simulink model "Recharge"  (R2020a)
settings: Solver=FixedStepAuto  StartTime=0.0  StopTime=10.0  FixedStep=1e-3  RelTol=1e-3  EnableMultiTasking=on
settings Model: ExtModeTrigDuration=5  Creator=WinnieTrandinh  LastModifiedBy=WinnieTrandinh
settings OptimizationCC: EnhancedBackFolding=on  PassReuseOutputArgsAs=Individual arguments  ZeroExternalMemoryAtStartup=off  ZeroInternalMemoryAtStartup=off  MaxStackSize=64  OptimizeBlockOrder=speed  DifferentSizesBufferReuse=on  OptimizationCustomize=off  EfficientTunableParamExpr=on
settings DebuggingCC: ParameterTunabilityLossMsg=error
settings HardwareCC: ProdBitPerPointer=32  ProdBitPerSizeT=32  ProdBitPerPtrDiffT=32  ProdLargestAtomicInteger=Long  ProdLargestAtomicFloat=Double  ProdWordSize=32  ProdHWDeviceType=ARM Compatible->ARM Cortex
settings SFSimCC: MATLABDynamicMemAlloc=off
settings RTWCC: SystemTargetFile=ert.tlc  HardwareBoard=NXP FRDM-K64F  TemplateMakefile=ert_default_tmf  Toolchain=GNU Tools for ARM Embedded Processors
settings CodeAppCC: ForceParamTrailComments=on  IgnoreCustomStorageClasses=off  OperatorAnnotations=on  SimulinkDataObjDesc=on  SFDataObjDesc=on  InsertBlockDesc=on

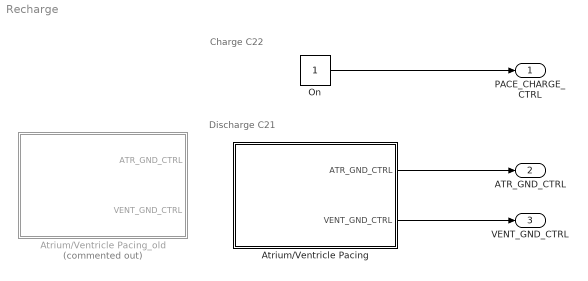
== system Recharge ==
  note: Discharge C21
  note: Charge C22
  Atrium/Ventricle Pacing : Subsystem
  Atrium/Ventricle Pacing_old : Subsystem  Commented=on  Variant=on
  On : Constant
  PACE_CHARGE_CTRL : Outport
  ATR_GND_CTRL : Outport  Port=2
  VENT_GND_CTRL : Outport  Port=3
  wires:
  On/1 -> PACE_CHARGE_CTRL/1
  Atrium/Ventricle Pacing/2(VENT_GND_CTRL) -> VENT_GND_CTRL/1
  Atrium/Ventricle Pacing/1(ATR_GND_CTRL) -> ATR_GND_CTRL/1

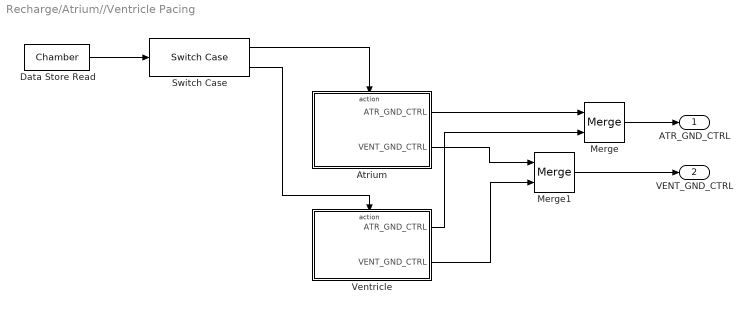
== system Recharge/Atrium//Ventricle Pacing ==
  Atrium : Subsystem  Priority=5  VariantControl=ATR_PACING
  Data Store Read : DataStoreRead  DataStoreName=Chamber
  Merge : Merge
  Merge1 : Merge
  Switch Case : SwitchCase  CaseConditions={1,2}  ShowDefaultCase=off
  Ventricle : Subsystem  Priority=5  VariantControl=VENT_PACING
  ATR_GND_CTRL : Outport
  VENT_GND_CTRL : Outport  Port=2
  wires:
  Atrium/1(ATR_GND_CTRL) -> Merge/1
  Ventricle/1(ATR_GND_CTRL) -> Merge/2
  Atrium/2(VENT_GND_CTRL) -> Merge1/1
  Ventricle/2(VENT_GND_CTRL) -> Merge1/2
  Merge1/1 -> VENT_GND_CTRL/1
  Merge/1 -> ATR_GND_CTRL/1
  Data Store Read/1 -> Switch Case/1
  Switch Case/1 -> Atrium/Action
  Switch Case/2 -> Ventricle/Action

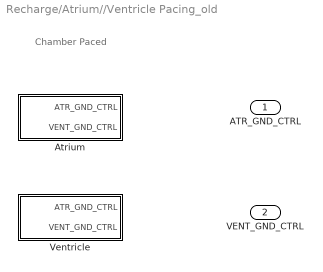
== system Recharge/Atrium//Ventricle Pacing_old ==
  note: Chamber Paced
  Atrium : Subsystem  Priority=5  VariantControl=ATR_PACING
  Ventricle : Subsystem  Priority=5  VariantControl=VENT_PACING
  ATR_GND_CTRL : Outport
  VENT_GND_CTRL : Outport  Port=2

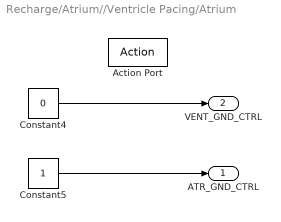
== system Recharge/Atrium//Ventricle Pacing/Atrium ==
  Action Port : ActionPort  ActionPortLabel=case [ 1 ]:
  Constant4 : Constant  Value=0
  Constant5 : Constant
  ATR_GND_CTRL : Outport
  VENT_GND_CTRL : Outport  Port=2
  wires:
  Constant5/1 -> ATR_GND_CTRL/1
  Constant4/1 -> VENT_GND_CTRL/1

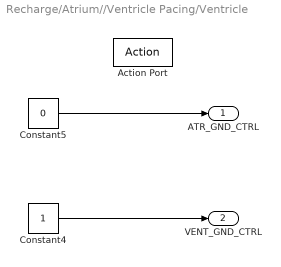
== system Recharge/Atrium//Ventricle Pacing/Ventricle ==
  Action Port : ActionPort  ActionPortLabel=case [ 2 ]:
  Constant4 : Constant
  Constant5 : Constant  Value=0
  ATR_GND_CTRL : Outport
  VENT_GND_CTRL : Outport  Port=2
  wires:
  Constant4/1 -> VENT_GND_CTRL/1
  Constant5/1 -> ATR_GND_CTRL/1

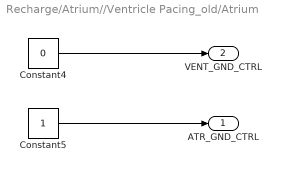
== system Recharge/Atrium//Ventricle Pacing_old/Atrium ==
  Constant4 : Constant  Value=0
  Constant5 : Constant
  ATR_GND_CTRL : Outport
  VENT_GND_CTRL : Outport  Port=2
  wires:
  Constant5/1 -> ATR_GND_CTRL/1
  Constant4/1 -> VENT_GND_CTRL/1

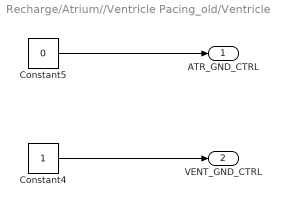
== system Recharge/Atrium//Ventricle Pacing_old/Ventricle ==
  Constant4 : Constant
  Constant5 : Constant  Value=0
  ATR_GND_CTRL : Outport
  VENT_GND_CTRL : Outport  Port=2
  wires:
  Constant4/1 -> VENT_GND_CTRL/1
  Constant5/1 -> ATR_GND_CTRL/1
